simulink model "tracking_model"  (R2017a)
settings: Solver=VariableStepAuto  StartTime=0.0  StopTime=10.0  RelTol=1e-3
undefined symbols (not defined in the file or in its folder): sys, x0
(part 14 of 14)

== matlab function tracking_model/Plant/Dynamic system/Mass_block/mass_tensor ==
  data: in1 input; M_matrix output
function M_matrix = Mass_matrix(in1)

%    This function was generated by the Symbolic Math Toolbox version 7.2.

%    12-Jan-2021 12:23:21



beta_ = in1(4,:);

th = in1(3,:);

t2 = beta_+th;

t3 = cos(t2);

t4 = cos(th);

t5 = sin(th);

t6 = sin(t2);

t16 = t3.*(1.0./5.0e2);

t7 = t4.*(-3.0./8.0e1)-t5.*(1.0./5.0e1)-t16;

t8 = t4.*(1.0./5.0e1);

t17 = t6.*(1.0./5.0e2);

t9 = t5.*(-3.0./8.0e1)+t8-t17;

t14 = t6.*(1.0./5.0e1);

t15 = t4.*(1.0./1.0e1);

t10 = -t14+t15;

t12 = t3.*(1.0./5.0e1);

t13 = t5.*(1.0./1.0e1);

t11 = t12+t13;

t18 = t3.*t11.*(1.0./5.0e2);

t19 = t14-t15;

t20 = t6.*t19.*(1.0./5.0e2);

t21 = t18+t20+1.0./5.0e1;

M_matrix = reshape([1.0,0.0,t7,-t16,0.0,0.0,0.0,0.0,1.0,t9,-t17,0.0,0.0,0.0,t7,t9,t4.^2.*4.5625e-3+t5.^2.*4.5625e-3+t10.^2.*(1.0./1.0e1)+t11.^2.*(1.0./1.0e1)+1.0./2.0e1,t21,0.0,0.0,0.0,t3.*(-1.0./5.0e2),t6.*(-1.0./5.0e2),t21,t3.^2.*4.0e-5+t6.^2.*4.0e-5+1.0./5.0e1,0.0,0.0,0.0,0.0,0.0,0.0,0.0,0.0,0.0,0.0,0.0,0.0,0.0,0.0,0.0,0.0,0.0,0.0,0.0,0.0,0.0,0.0,0.0,0.0],[7,7]);

end

== matlab function tracking_model/Plant/Dynamic system/Auxiliary_matrices/C_matrix ==
  data: in1 input; C output
function C = ConstraintMatrix(in1)

%    This function was generated by the Symbolic Math Toolbox version 7.2.

%    12-Jan-2021 12:23:20



beta_ = in1(4,:);

th = in1(3,:);

t2 = cos(beta_);

t3 = sin(beta_);

t4 = t2.*(1.0./1.0e1);

t5 = t3.*7.5e-2i;

t6 = t4+t5;

t7 = t2.^2;

t8 = t7.*(1.0./1.0e2);

t9 = t3.^2;

t10 = t9.*5.625e-3;

t11 = t8+t10;

t12 = 1.0./sqrt(t11);

t13 = angle(t6);

t14 = beta_-t13;

t15 = cos(t14);

t16 = t13+th;

t17 = sin(t16);

t18 = abs(t6);

t19 = 1.0./t18;

t20 = t2.*(2.0./5.0);

t21 = t3.*(1.0./5.0);

C = reshape([0.0,0.0,0.0,1.0,0.0,0.0,0.0,cos(beta_+th).*(1.0./5.0e1),(t12.*cos(beta_+t13+th.*2.0).*(-2.0e-4)-t12.*t15.*2.0e-4+t12.*sin(beta_-t13+th).*1.5e-4+t12.*sin(beta_+t13+th).*1.5e-4+1.0./2.5e2)./(t12.*t17.*(1.0./5.0e1)+t2.*t12.*t19.*1.5e-3),(t12.*t15.*(1.0./5.0e2)-1.0./5.0e1)./(t12.*t17.*(1.0./1.0e2)+t2.*t12.*t19.*7.5e-4),0.0,t20+t21,t20-t21,1.0],[7,2]);

end

== matlab function tracking_model/trajectory_function ==
  data: t input; trajs output
function trajs = TrajectoryGenerator(t)

%    This function was generated by the Symbolic Math Toolbox version 7.2.

%    10-Jan-2021 16:30:39



trajs = [cos(t.*1.0e1);sin(t.*1.0e1).*-1.0e1;cos(t.*1.0e1).*-1.0e2;sin(t.*1.0e1);cos(t.*1.0e1).*1.0e1;sin(t.*1.0e1).*-1.0e2;t.*1.0e1;1.0e1;0.0];

end

== matlab function tracking_model/Plant/Dynamic system/Efforts/Constrained_efforts ==
  data: in1 input; fs output; in2 input
function fs = ConstrainedEffort(in1,in2)

%    This function was generated by the Symbolic Math Toolbox version 7.2.

%    12-Jan-2021 12:23:28



beta_ = in1(4,:);

p1 = in1(8,:);

p2 = in1(9,:);

tau_f = in2(1,:);

tau_l = in2(3,:);

tau_r = in2(2,:);

th = in1(3,:);

t2 = beta_+th;

t3 = cos(t2);

t4 = cos(beta_);

t5 = sin(beta_);

t6 = t4.*(1.0./1.0e1);

t7 = t5.*7.5e-2i;

t8 = t6+t7;

t9 = angle(t8);

t10 = t4.^2;

t11 = t10.*(1.0./1.0e2);

t12 = t5.^2;

t13 = t12.*5.625e-3;

t14 = t11+t13;

t15 = 1.0./sqrt(t14);

t16 = t9+th;

t17 = sin(t16);

t18 = abs(t8);

t19 = 1.0./t18;

t20 = t9.*-1.0;

t21 = beta_+t20;

t22 = cos(t21);

t23 = t15.*t22.*(1.0./1.0e1);

t24 = t23-1.0;

t25 = t15.*t17.*(1.0./1.0e2);

t26 = t4.*t15.*t19.*7.5e-4;

t27 = t25+t26;

t28 = 1.0./t27;

t29 = sin(t2);

t30 = p1.*t29.*(1.0./5.0e1);

t31 = p2.*t24.*t28.*t29.*4.0e-4;

t32 = p1.*t3.*(1.0./5.0e1);

t33 = p2.*t3.*t24.*t28.*4.0e-4;

t34 = t15.*t17.*2.0e-2;

t35 = t4.*t15.*t19.*1.5e-3;

t36 = t34+t35;

t37 = 1.0./t36;

t38 = beta_+t9+th;

t39 = sin(t38);

t40 = t15.*t39.*(3.0./4.0e2);

t41 = t15.*t22.*-1.0e-2;

t42 = th.*2.0;

t43 = beta_+t9+t42;

t44 = cos(t43);

t45 = t15.*t44.*-1.0e-2;

t46 = beta_+t20+th;

t47 = sin(t46);

t48 = t15.*t47.*(3.0./4.0e2);

t49 = t40+t41+t45+t48+2.0e-1;

t50 = p2.*t37.*t49.*-2.0e-2;

t51 = cos(th);

t52 = p2.*t24.*t28.*t51.*-2.0e-3;

t53 = t30+t31+t50+t52;

t54 = p2.*t3.*-2.0e-2;

t55 = sin(th);

t56 = p2.*t24.*t28.*t55.*(1.0./5.0e2);

t57 = t32+t33+t54+t56;

t58 = t32+t33;

t59 = t30+t31;

t60 = t3.*t53.*(1.0./5.0e2);

t61 = t29.*t57.*-2.0e-3;

t62 = t4.*(1.0./5.0);

t63 = t5.*(1.0./1.0e1);

t64 = t32+t33+t56;

t65 = t30+t31+t52;

t66 = t3.*(1.0./5.0e1);

t67 = t55.*(1.0./1.0e1);

t68 = t66+t67;

t69 = t29.*(1.0./5.0e1);

t70 = p2.*t3.*(1.0./5.0e1);

t71 = p2.*t37.*t49.*(1.0./5.0e1);

t72 = t51.*1.0e-1;

t73 = t69-t72;

t76 = p2.*t24.*t28.*t51.*1.0e-3;

t74 = -t76;

t75 = t70+t74;

t77 = p2.*t24.*t28.*t55.*-2.0e-3;

t78 = t70+t77;

t79 = p2.*t24.*t28.*t51.*(1.0./5.0e2);

t80 = t71+t79;

t81 = p2.*t24.*t28.*t51.*-1.5e-3;

t82 = t70+t81;

t85 = p2.*t24.*t28.*t55.*1.0e-3;

t83 = -t85;

t84 = t71+t83;

t86 = p2.*t24.*t28.*t55.*-1.5e-3;

t87 = t71+t86;

fs = [tau_f+t53.*t58.*1.0e-1-t57.*t59.*(1.0./1.0e1)-p1.*(t60+t61-t3.*t59.*2.0e-3+t29.*t58.*(1.0./5.0e2))-p2.*t24.*t28.*(t60+t61-t3.*t65.*2.0e-3+t29.*t64.*(1.0./5.0e2)).*(1.0./5.0e1);tau_r.*(t62+t63).*2.0+tau_l.*(t62-t63).*2.0-t3.*(p1.*(p1.*t29.*4.0e-2+p2.*t24.*t28.*t29.*8.0e-4).*5.0e-2+p2.*t24.*t28.*(p1.*t29.*2.0e-3+p2.*t24.*t28.*t29.*4.0e-5-p2.*t24.*t28.*t51.*4.0e-4+p2.*t24.*t28.*t55.*7.5e-4).*(1.0./5.0e1)).*(1.0./5.0e1)+t37.*t49.*(p1.*(p1.*t3.*4.0e-2+p2.*t3.*t24.*t28.*8.0e-4).*5.0e-2+p2.*t24.*t28.*(p1.*t3.*2.0e-3+p2.*t3.*t24.*t28.*4.0e-5+p2.*t24.*t28.*t51.*7.5e-4+p2.*t24.*t28.*t55.*4.0e-4).*(1.0./5.0e1)).*2.0e-2-t24.*t28.*(t53.*t64.*(-1.0./1.0e1)+t57.*t65.*1.0e-1+p1.*(t3.*t53.*2.0e-3-t29.*t57.*(1.0./5.0e2)-t59.*t68.*(1.0./1.0e1)+t58.*t73.*1.0e-1)-p2.*t24.*t28.*(t55.*(t70+p2.*t24.*t28.*t51.*1.0e-3).*7.5e-3-t51.*(t71+p2.*t24.*t28.*t55.*1.0e-3).*7.5e-3-t53.*t68.*1.0e-1+t51.*t78.*(1.0./1.0e2)-t55.*t75.*7.5e-3+t57.*t73.*(1.0./1.0e1)+t65.*t68.*(1.0./1.0e1)+t51.*t84.*7.5e-3+t55.*t80.*(1.0./1.0e2)-t55.*t82.*3.75e-2-t64.*t73.*1.0e-1+t51.*t87.*(3.0./8.0e1)).*(1.0./5.0e1)+p2.*t24.*t28.*t55.*(t70+t76).*1.5e-4-p2.*t24.*t28.*t51.*(t71+t85).*1.5e-4+p2.*t24.*t28.*t51.*t78.*2.0e-4-p2.*t24.*t28.*t55.*t75.*1.5e-4+p2.*t24.*t28.*t51.*t84.*1.5e-4+p2.*t24.*t28.*t55.*t80.*2.0e-4-p2.*t24.*t28.*t55.*t82.*7.5e-4+p2.*t24.*t28.*t51.*t87.*7.5e-4).*2.0e-2];

end

== matlab function tracking_model/Plant/Dynamic system/Mass_block/H ==
  data: C_matrix input; H output; M input
function H = ConstrinedMassMatrix(C_matrix, M)
% MASSMATRIX
%    This function was generated by the Symbolic Math Toolbox version 7.2.
%    16-Oct-2020 11:55:07

    H = C_matrix'*M*C_matrix;
end

== matlab function tracking_model/Plant/Dynamic system/Mass_block/invH ==
  data: matrix input; inv_matrix output
function inv_matrix = matrix_inverse(matrix)
% MASSMATRIX
%    This function was generated by the Symbolic Math Toolbox version 7.2.
%    16-Oct-2020 11:55:07

    inv_matrix = inv(matrix);
end

== matlab function tracking_model/Plant/Dynamic system/Auxiliary_matrices/C_p ==
  data: in1 input; qp output
function qp = KinematicVector(in1)

%    This function was generated by the Symbolic Math Toolbox version 7.2.

%    12-Jan-2021 12:23:20



beta_ = in1(4,:);

p1 = in1(8,:);

p2 = in1(9,:);

th = in1(3,:);

t2 = cos(beta_);

t3 = sin(beta_);

t4 = t2.*(1.0./1.0e1);

t5 = t3.*7.5e-2i;

t6 = t4+t5;

t7 = t2.^2;

t8 = t7.*(1.0./1.0e2);

t9 = t3.^2;

t10 = t9.*5.625e-3;

t11 = t8+t10;

t12 = 1.0./sqrt(t11);

t13 = angle(t6);

t14 = beta_-t13;

t15 = cos(t14);

t16 = t13+th;

t17 = sin(t16);

t18 = abs(t6);

t19 = 1.0./t18;

t20 = t2.*(1.0./5.0);

t21 = t3.*(1.0./1.0e1);

qp = [p2.*cos(beta_+th).*(1.0./5.0e1);(p2.*(t12.*cos(beta_+t13+th.*2.0).*(-1.0./1.0e2)-t12.*t15.*(1.0./1.0e2)+t12.*sin(beta_-t13+th).*(3.0./4.0e2)+t12.*sin(beta_+t13+th).*(3.0./4.0e2)+1.0./5.0).*(1.0./5.0e1))./(t12.*t17.*(1.0./5.0e1)+t2.*t12.*t19.*1.5e-3);(p2.*(t12.*t15.*(1.0./1.0e1)-1.0).*(1.0./5.0e1))./(t12.*t17.*(1.0./1.0e2)+t2.*t12.*t19.*7.5e-4);p1;p2.*(t20+t21).*2.0;p2.*(t20-t21).*2.0;p2];

end
